simulink model "Subsystem0"  (R2020a)
settings: Solver=FixedStepAuto  StartTime=0.0  StopTime=10.0  FixedStep=0.2  RelTol=1e-3
settings Model: Creator=Riyansh  LastModifiedBy=Riyansh
settings DataIOCC: SaveOutput=off  SaveTime=off

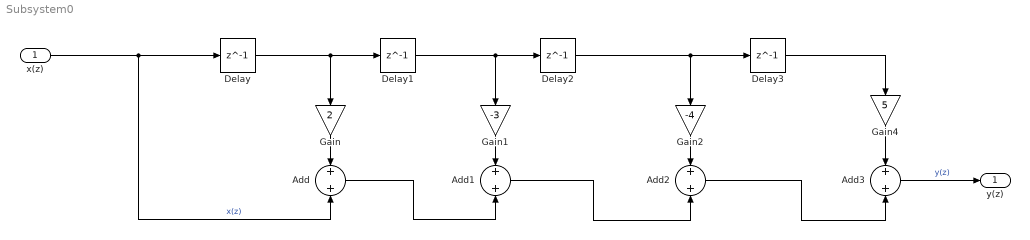
== system Subsystem0 ==
  x(z) : Inport  OutDataTypeStr=double  PortDimensions=1  SampleTime=[0.20000000000000001,0]
  Add{,1..3} (4 alike) : Sum
  Delay{,1..3} (4 alike) : Delay  DelayLength=1  InitialCondition=0
  Gain : Gain  Gain=2
  Gain1 : Gain  Gain=-3
  Gain2 : Gain  Gain=-4
  Gain4 : Gain  Gain=5
  y(z) : Outport  OutDataTypeStr=double  PortDimensions=1  SampleTime=[0.20000000000000001,0]
  wires:
  Gain/1 -> Add/1
  Delay/1 -> Delay1/1, Gain/1
  Gain1/1 -> Add1/1
  Delay1/1 -> Delay2/1, Gain1/1
  Delay2/1 -> Delay3/1, Gain2/1
  Gain4/1 -> Add3/1
  Add/1 -> Add1/2
  Add2/1 -> Add3/2
  Add1/1 -> Add2/2
  Gain2/1 -> Add2/1
  Delay3/1 -> Gain4/1
  x(z)/1 -> Add/2, Delay/1  "x(z)"
  Add3/1 -> y(z)/1  "y(z)"
